simulink model "Problem4_2ndWeek"  (R2020b)
settings: Solver=VariableStepAuto  StartTime=0.0  StopTime=0.2  RelTol=1e-3
model workspace (MAT data in the model file):
  J = Simulink.Parameter
  J.Value = 3.2284e-06
  J.DataType = 'auto'
  J.Dimensions = [1 1]
  K = Simulink.Parameter
  K.Value = 0.0274
  K.DataType = 'auto'
  K.Dimensions = [1 1]
  Kd = Simulink.Parameter
  Kd.Value = 0.15
  Kd.DataType = 'auto'
  Kd.Dimensions = [1 1]
  Ki = Simulink.Parameter
  Ki.Value = 620
  Ki.DataType = 'auto'
  Ki.Dimensions = [1 1]
  Kp = Simulink.Parameter
  Kp.Value = 19
  Kp.DataType = 'auto'
  Kp.Dimensions = [1 1]
  L = Simulink.Parameter
  L.Value = 2.75e-06
  L.DataType = 'auto'
  L.Dimensions = [1 1]
  N = Simulink.Parameter
  N.Value = 10000
  N.DataType = 'auto'
  N.Dimensions = [1 1]
  R = Simulink.Parameter
  R.Value = 4
  R.DataType = 'auto'
  R.Dimensions = [1 1]
  b = Simulink.Parameter
  b.Value = 3.5077e-06
  b.DataType = 'auto'
  b.Dimensions = [1 1]
settings Model: Creator=hp  LastModifiedBy=hp

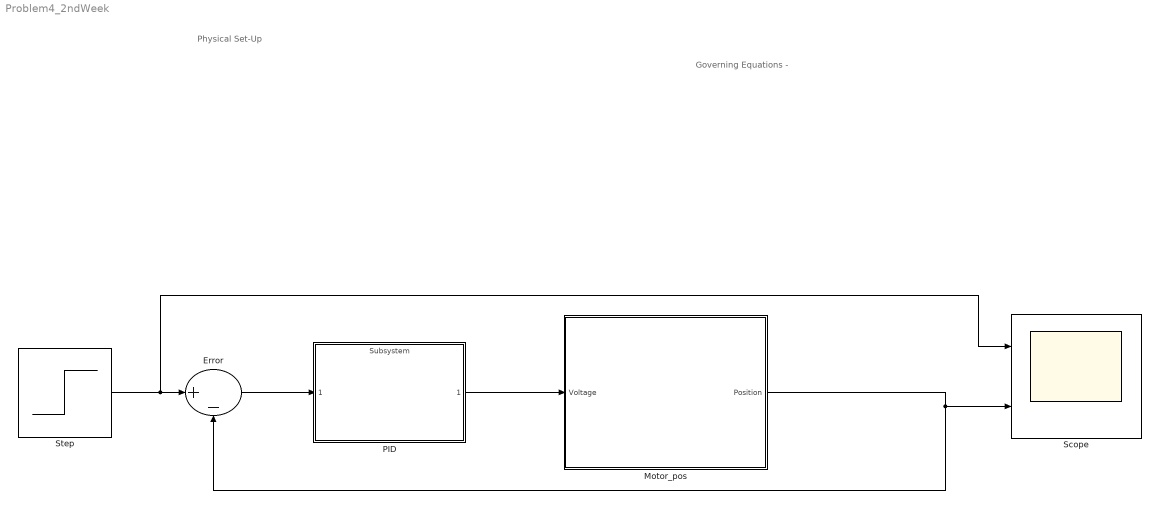
== system Problem4_2ndWeek ==
  note: Governing Equations -
  note: Physical Set-Up
  Error : Sum  Inputs=|+-
  Motor_pos : Subsystem
  PID : ModelReference  ModelNameDialog=Subsystem  SimulationMode=Normal  ModelReferenceVersion=1.3
  Scope : Scope  NumInputPorts=2
  Step : Step  Time=0  SampleTime=0
  wires:
  PID/1 -> Motor_pos/1(Voltage)
  Error/1 -> PID/1
  Motor_pos/1(Position) -> Scope/2, Error/2
  Step/1 -> Scope/1, Error/1

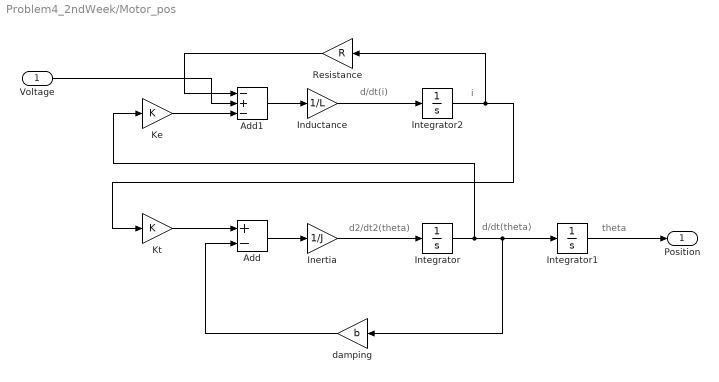
== system Problem4_2ndWeek/Motor_pos ==
  note: i
  note: d/dt(i)
  note: d2/dt2(theta)
  note: d/dt(theta)
  note: theta
  Voltage : Inport
  Add : Sum  Inputs=+-
  Add1 : Sum  Inputs=-+-
  Inductance : Gain  Gain=1/L
  Inertia : Gain  Gain=1/J
  Integrator : Integrator
  Integrator1 : Integrator
  Integrator2 : Integrator
  Ke : Gain  Gain=K
  Kt : Gain  Gain=K
  Resistance : Gain  Gain=R
  damping : Gain  Gain=b
  Position : Outport
  wires:
  Inertia/1 -> Integrator/1
  Inductance/1 -> Integrator2/1
  Integrator2/1 -> Resistance/1, Kt/1
  Integrator/1 -> Ke/1, damping/1, Integrator1/1
  Integrator1/1 -> Position/1
  Voltage/1 -> Add1/2
  Add/1 -> Inertia/1
  damping/1 -> Add/2
  Kt/1 -> Add/1
  Resistance/1 -> Add1/1
  Ke/1 -> Add1/3
  Add1/1 -> Inductance/1
